simulink model "reseau_alarm"  (R2017a)
settings: Solver=VariableStepAuto  StartTime=0.0  StopTime=1  RelTol=1e-3
libraries: commrandsrc3 x5
settings Model: Creator=floriant  LastModifiedBy=floriant

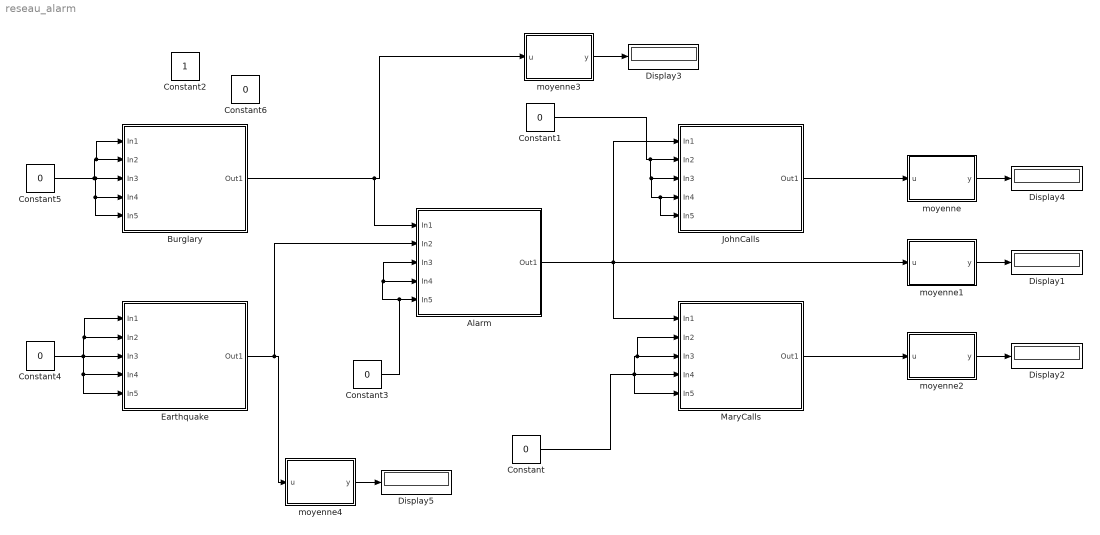
== system reseau_alarm ==
  Alarm : Subsystem
  Burglary : Subsystem
  Constant{,1,3..6} (6 alike) : Constant  Value=0  OutDataTypeStr=boolean
  Constant2 : Constant  OutDataTypeStr=boolean
  Display{1..5} (5 alike) : Display
  Earthquake : Subsystem
  JohnCalls : Subsystem
  MaryCalls : Subsystem
  moyenne : MATLAB Function  TreatAsAtomicUnit=on
  moyenne1 : MATLAB Function  TreatAsAtomicUnit=on
  moyenne2 : MATLAB Function  TreatAsAtomicUnit=on
  moyenne3 : MATLAB Function  TreatAsAtomicUnit=on
  moyenne4 : MATLAB Function  TreatAsAtomicUnit=on
  wires:
  moyenne/1(y) -> Display4/1
  JohnCalls/1(Out1) -> moyenne/1(u)
  moyenne1/1(y) -> Display1/1
  Alarm/1(Out1) -> moyenne1/1(u), JohnCalls/1(In1), MaryCalls/1(In1)
  Constant/1 -> MaryCalls/2(In2), MaryCalls/3(In3), MaryCalls/4(In4), MaryCalls/5(In5)
  Constant1/1 -> JohnCalls/5(In5), JohnCalls/4(In4), JohnCalls/3(In3), JohnCalls/2(In2)
  Earthquake/1(Out1) -> Alarm/2(In2), moyenne4/1(u)
  Constant4/1 -> Earthquake/5(In5), Earthquake/4(In4), Earthquake/3(In3), Earthquake/1(In1), Earthquake/2(In2)
  Constant5/1 -> Burglary/1(In1), Burglary/2(In2), Burglary/4(In4), Burglary/5(In5), Burglary/3(In3)
  Burglary/1(Out1) -> Alarm/1(In1), moyenne3/1(u)
  Constant3/1 -> Alarm/4(In4), Alarm/3(In3), Alarm/5(In5)
  MaryCalls/1(Out1) -> moyenne2/1(u)
  moyenne2/1(y) -> Display2/1
  moyenne3/1(y) -> Display3/1
  moyenne4/1(y) -> Display5/1

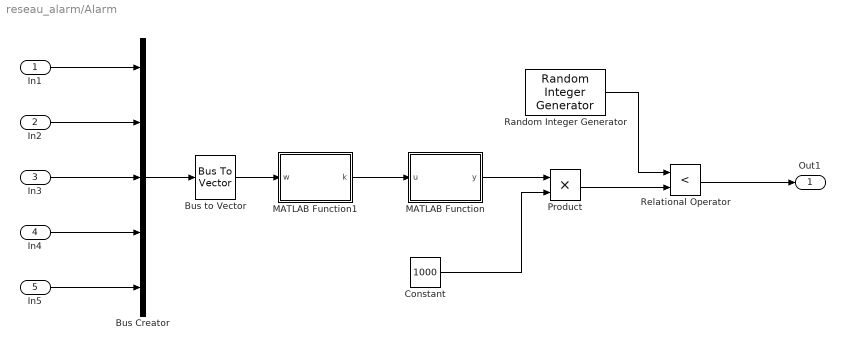
== system reseau_alarm/Alarm ==
  In1 : Inport  OutDataTypeStr=boolean
  In2 : Inport  Port=2  OutDataTypeStr=boolean
  In3 : Inport  Port=3  OutDataTypeStr=boolean
  In4 : Inport  Port=4  OutDataTypeStr=boolean
  In5 : Inport  Port=5  OutDataTypeStr=boolean
  Bus Creator : BusCreator  Inputs=5
  Bus to Vector : BusToVector
  Constant : Constant  Value=1000
  MATLAB Function : MATLAB Function  TreatAsAtomicUnit=on
  MATLAB Function1 : MATLAB Function  TreatAsAtomicUnit=on
  Product : Product
  Random Integer Generator : commrandsrc3/Random Integer Generator  SetSize=1000  SeedSource=Auto  Seed=0  SampleTime=1e-6  SamplesPerFrame=1  OutputDataType=uint16  SimulateUsing=Interpreted execution
  Relational Operator : RelationalOperator  Operator=<  OutDataTypeStr=boolean  RndMeth=Simplest
  Out1 : Outport
  wires:
  In5/1 -> Bus Creator/5
  In4/1 -> Bus Creator/4
  Bus to Vector/1 -> MATLAB Function1/1(w)
  Constant/1 -> Product/2
  Random Integer Generator/1 -> Relational Operator/1
  In2/1 -> Bus Creator/2
  MATLAB Function1/1(k) -> MATLAB Function/1(u)
  Product/1 -> Relational Operator/2
  MATLAB Function/1(y) -> Product/1
  In1/1 -> Bus Creator/1
  In3/1 -> Bus Creator/3
  Bus Creator/1 -> Bus to Vector/1
  Relational Operator/1 -> Out1/1

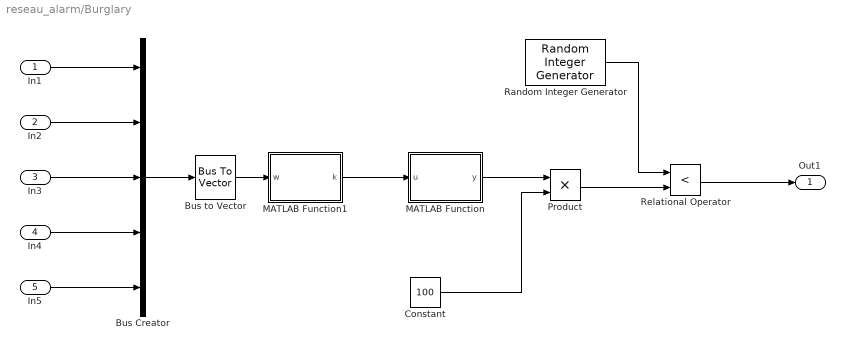
== system reseau_alarm/Burglary ==
  In1 : Inport  OutDataTypeStr=boolean
  In2 : Inport  Port=2  OutDataTypeStr=boolean
  In3 : Inport  Port=3  OutDataTypeStr=boolean
  In4 : Inport  Port=4  OutDataTypeStr=boolean
  In5 : Inport  Port=5  OutDataTypeStr=boolean
  Bus Creator : BusCreator  Inputs=5
  Bus to Vector : BusToVector
  Constant : Constant  Value=100
  MATLAB Function : MATLAB Function  TreatAsAtomicUnit=on
  MATLAB Function1 : MATLAB Function  TreatAsAtomicUnit=on
  Product : Product
  Random Integer Generator : commrandsrc3/Random Integer Generator  SetSize=100  SeedSource=Auto  Seed=0  SampleTime=1e-6  SamplesPerFrame=1  OutputDataType=uint8  SimulateUsing=Interpreted execution
  Relational Operator : RelationalOperator  Operator=<  OutDataTypeStr=boolean  RndMeth=Simplest
  Out1 : Outport
  wires:
  In5/1 -> Bus Creator/5
  In4/1 -> Bus Creator/4
  Bus to Vector/1 -> MATLAB Function1/1(w)
  Constant/1 -> Product/2
  Random Integer Generator/1 -> Relational Operator/1
  In2/1 -> Bus Creator/2
  MATLAB Function1/1(k) -> MATLAB Function/1(u)
  Product/1 -> Relational Operator/2
  MATLAB Function/1(y) -> Product/1
  In1/1 -> Bus Creator/1
  In3/1 -> Bus Creator/3
  Bus Creator/1 -> Bus to Vector/1
  Relational Operator/1 -> Out1/1

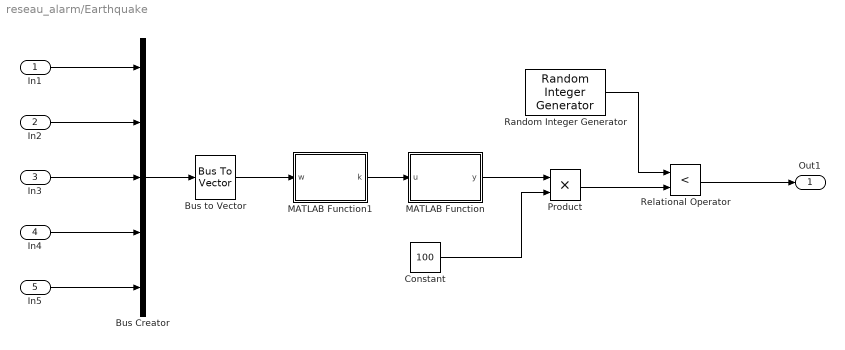
== system reseau_alarm/Earthquake ==
  In1 : Inport  OutDataTypeStr=boolean
  In2 : Inport  Port=2  OutDataTypeStr=boolean
  In3 : Inport  Port=3  OutDataTypeStr=boolean
  In4 : Inport  Port=4  OutDataTypeStr=boolean
  In5 : Inport  Port=5  OutDataTypeStr=boolean
  Bus Creator : BusCreator  Inputs=5
  Bus to Vector : BusToVector
  Constant : Constant  Value=100
  MATLAB Function : MATLAB Function  TreatAsAtomicUnit=on
  MATLAB Function1 : MATLAB Function  TreatAsAtomicUnit=on
  Product : Product
  Random Integer Generator : commrandsrc3/Random Integer Generator  SetSize=100  SeedSource=Auto  Seed=0  SampleTime=1e-6  SamplesPerFrame=1  OutputDataType=uint8  SimulateUsing=Interpreted execution
  Relational Operator : RelationalOperator  Operator=<  OutDataTypeStr=boolean  RndMeth=Simplest
  Out1 : Outport
  wires:
  In5/1 -> Bus Creator/5
  In4/1 -> Bus Creator/4
  Bus to Vector/1 -> MATLAB Function1/1(w)
  Constant/1 -> Product/2
  Random Integer Generator/1 -> Relational Operator/1
  In2/1 -> Bus Creator/2
  MATLAB Function1/1(k) -> MATLAB Function/1(u)
  Product/1 -> Relational Operator/2
  MATLAB Function/1(y) -> Product/1
  In1/1 -> Bus Creator/1
  In3/1 -> Bus Creator/3
  Bus Creator/1 -> Bus to Vector/1
  Relational Operator/1 -> Out1/1

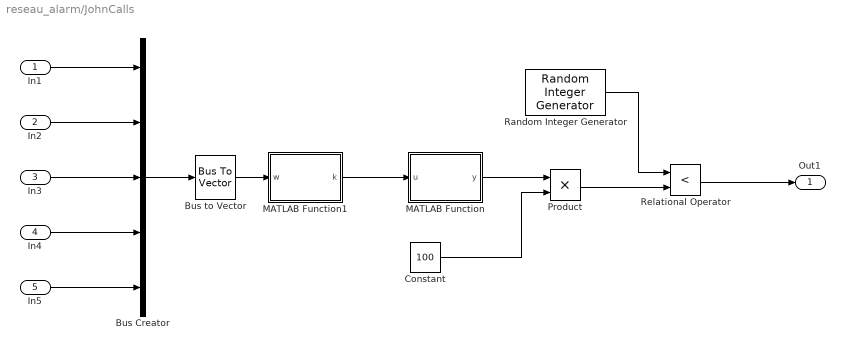
== system reseau_alarm/JohnCalls ==
  In1 : Inport  OutDataTypeStr=boolean
  In2 : Inport  Port=2  OutDataTypeStr=boolean
  In3 : Inport  Port=3  OutDataTypeStr=boolean
  In4 : Inport  Port=4  OutDataTypeStr=boolean
  In5 : Inport  Port=5  OutDataTypeStr=boolean
  Bus Creator : BusCreator  Inputs=5
  Bus to Vector : BusToVector
  Constant : Constant  Value=100
  MATLAB Function : MATLAB Function  TreatAsAtomicUnit=on
  MATLAB Function1 : MATLAB Function  TreatAsAtomicUnit=on
  Product : Product
  Random Integer Generator : commrandsrc3/Random Integer Generator  SetSize=100  SeedSource=Auto  Seed=0  SampleTime=1e-6  SamplesPerFrame=1  OutputDataType=uint8  SimulateUsing=Interpreted execution
  Relational Operator : RelationalOperator  Operator=<  OutDataTypeStr=boolean  RndMeth=Simplest
  Out1 : Outport
  wires:
  In5/1 -> Bus Creator/5
  In4/1 -> Bus Creator/4
  Bus to Vector/1 -> MATLAB Function1/1(w)
  Constant/1 -> Product/2
  Random Integer Generator/1 -> Relational Operator/1
  In2/1 -> Bus Creator/2
  MATLAB Function1/1(k) -> MATLAB Function/1(u)
  Product/1 -> Relational Operator/2
  MATLAB Function/1(y) -> Product/1
  In1/1 -> Bus Creator/1
  In3/1 -> Bus Creator/3
  Bus Creator/1 -> Bus to Vector/1
  Relational Operator/1 -> Out1/1

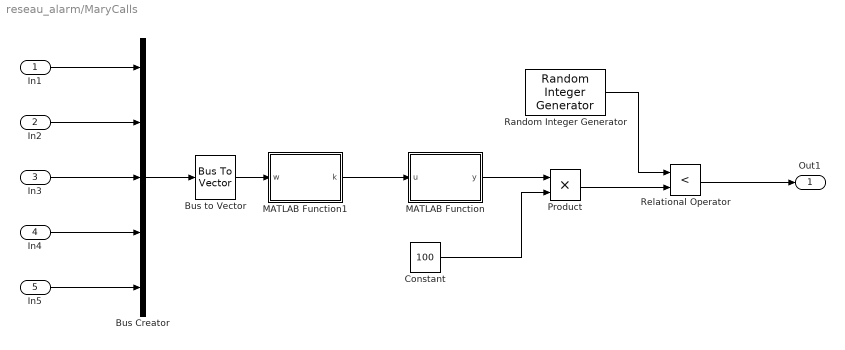
== system reseau_alarm/MaryCalls ==
  In1 : Inport  OutDataTypeStr=boolean
  In2 : Inport  Port=2  OutDataTypeStr=boolean
  In3 : Inport  Port=3  OutDataTypeStr=boolean
  In4 : Inport  Port=4  OutDataTypeStr=boolean
  In5 : Inport  Port=5  OutDataTypeStr=boolean
  Bus Creator : BusCreator  Inputs=5
  Bus to Vector : BusToVector
  Constant : Constant  Value=100
  MATLAB Function : MATLAB Function  TreatAsAtomicUnit=on
  MATLAB Function1 : MATLAB Function  TreatAsAtomicUnit=on
  Product : Product
  Random Integer Generator : commrandsrc3/Random Integer Generator  SetSize=100  SeedSource=Auto  Seed=0  SampleTime=1e-6  SamplesPerFrame=1  OutputDataType=uint8  SimulateUsing=Interpreted execution
  Relational Operator : RelationalOperator  Operator=<  OutDataTypeStr=boolean  RndMeth=Simplest
  Out1 : Outport
  wires:
  In5/1 -> Bus Creator/5
  In4/1 -> Bus Creator/4
  Bus to Vector/1 -> MATLAB Function1/1(w)
  Constant/1 -> Product/2
  Random Integer Generator/1 -> Relational Operator/1
  In2/1 -> Bus Creator/2
  MATLAB Function1/1(k) -> MATLAB Function/1(u)
  Product/1 -> Relational Operator/2
  MATLAB Function/1(y) -> Product/1
  In1/1 -> Bus Creator/1
  In3/1 -> Bus Creator/3
  Bus Creator/1 -> Bus to Vector/1
  Relational Operator/1 -> Out1/1

== matlab function reseau_alarm/moyenne ==
  data: u input; y output
function y = fcn(u)
persistent nb_one total
if isempty(nb_one)
    nb_one=0;
end
if isempty(total)
    total=0;
end
if u==1
    nb_one = nb_one+1;
end
total = total +1;

y=nb_one/total;

== matlab function reseau_alarm/Alarm/MATLAB Function ==
  data: u input; y output
function y = fcn(u)

MEM =[0.001;0.94;0.29;0.95];

y=MEM(u+1);

== matlab function reseau_alarm/Alarm/MATLAB Function1 ==
  data: w input; k output
function k = fcn(w)
out =0;
    if w(1)==1
        out = out + 1;
    end
    if w(2)==1
        out = out + 2;
    end
    if w(3)==1
        out = out + 4;
    end
    if w(4)==1
        out = out + 8;
    end
    if w(5)==1
        out = out + 16;
    end
k=out;

== matlab function reseau_alarm/Burglary/MATLAB Function ==
  data: u input; y output
function y = fcn(u)

MEM =[0.01];

y=MEM(u+1);

== matlab function reseau_alarm/Burglary/MATLAB Function1 ==
  data: w input; k output
function k = fcn(w)
out =0;
    if w(1)==1
        out = out + 1;
    end
    if w(2)==1
        out = out + 2;
    end
    if w(3)==1
        out = out + 4;
    end
    if w(4)==1
        out = out + 8;
    end
    if w(5)==1
        out = out + 16;
    end
k=out;

== matlab function reseau_alarm/Earthquake/MATLAB Function ==
  data: u input; y output
function y = fcn(u)

MEM =[0.02];

y=MEM(u+1);

== matlab function reseau_alarm/Earthquake/MATLAB Function1 ==
  data: w input; k output
function k = fcn(w)
out =0;
    if w(1)==1
        out = out + 1;
    end
    if w(2)==1
        out = out + 2;
    end
    if w(3)==1
        out = out + 4;
    end
    if w(4)==1
        out = out + 8;
    end
    if w(5)==1
        out = out + 16;
    end
k=out;

== matlab function reseau_alarm/JohnCalls/MATLAB Function ==
  data: u input; y output
function y = fcn(u)

MEM =[0.05;0.9];

y=MEM(u+1);

== matlab function reseau_alarm/JohnCalls/MATLAB Function1 ==
  data: w input; k output
function k = fcn(w)
out =0;
    if w(1)==1
        out = out + 1;
    end
    if w(2)==1
        out = out + 2;
    end
    if w(3)==1
        out = out + 4;
    end
    if w(4)==1
        out = out + 8;
    end
    if w(5)==1
        out = out + 16;
    end
k=out;

== matlab function reseau_alarm/MaryCalls/MATLAB Function ==
  data: u input; y output
function y = fcn(u)

MEM =[0.01;0.7];

y=MEM(u+1);

== matlab function reseau_alarm/MaryCalls/MATLAB Function1 ==
  data: w input; k output
function k = fcn(w)
out =0;
    if w(1)==1
        out = out + 1;
    end
    if w(2)==1
        out = out + 2;
    end
    if w(3)==1
        out = out + 4;
    end
    if w(4)==1
        out = out + 8;
    end
    if w(5)==1
        out = out + 16;
    end
k=out;

== matlab function reseau_alarm/moyenne1 ==
  data: u input; y output
function y = fcn(u)
persistent nb_one total
if isempty(nb_one)
    nb_one=0;
end
if isempty(total)
    total=0;
end
if u==1
    nb_one = nb_one+1;
end
total = total +1;

y=nb_one/total;

== matlab function reseau_alarm/moyenne2 ==
  data: u input; y output
function y = fcn(u)
persistent nb_one total
if isempty(nb_one)
    nb_one=0;
end
if isempty(total)
    total=0;
end
if u==1
    nb_one = nb_one+1;
end
total = total +1;

y=nb_one/total;

== matlab function reseau_alarm/moyenne3 ==
  data: u input; y output
function y = fcn(u)
persistent nb_one total
if isempty(nb_one)
    nb_one=0;
end
if isempty(total)
    total=0;
end
if u==1
    nb_one = nb_one+1;
end
total = total +1;

y=nb_one/total;

== matlab function reseau_alarm/moyenne4 ==
  data: u input; y output
function y = fcn(u)
persistent nb_one total
if isempty(nb_one)
    nb_one=0;
end
if isempty(total)
    total=0;
end
if u==1
    nb_one = nb_one+1;
end
total = total +1;

y=nb_one/total;
